simulink model "Calib_optitrack"  (R2024a)
settings: Solver=VariableStepAuto  StartTime=0.0  StopTime=10.0  RelTol=1e-3
libraries: robotcorelib x2
settings Model: Creator=user  LastModifiedBy=user

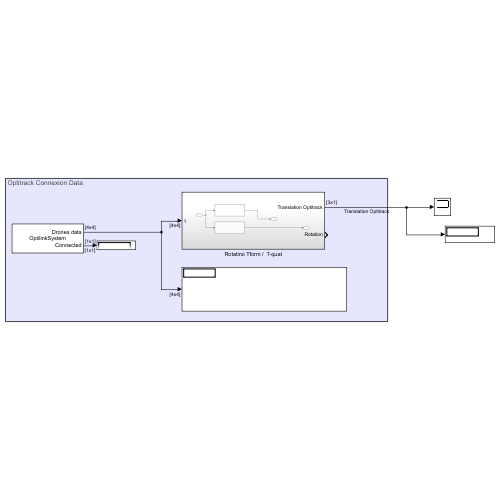
[thumbnail: Simulink's stored preview of the top-level diagram]
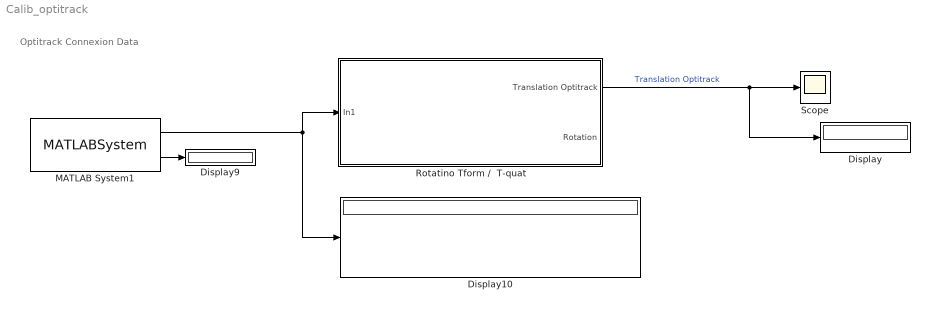
== system Calib_optitrack ==
  note: Optitrack Connexion Data
  Display : Display
  Display10 : Display
  Display9 : Display
  MATLAB System1 : MATLABSystem  System=OptilinkSystem  HostIP=127.0.0.1  ClientIP=127.0.0.1  SimulateUsing=Interpreted execution
      mask Type: OptilinkSystem
      mask Display:
      | disp('OptilinkSystem');
      | port_label('output',1,'Drones data');
      | port_label('output',2,'Connected');
  Rotatino Tform /  T-quat : Subsystem
  Scope : Scope
  wires:
  MATLAB System1/2 -> Display9/1
  Rotatino Tform /  T-quat/1(Translation Optitrack) -> Display/1, Scope/1  "Translation Optitrack"
  MATLAB System1/1 -> Rotatino Tform /  T-quat/1(In1), Display10/1

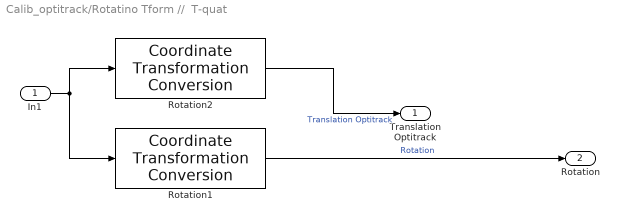
== system Calib_optitrack/Rotatino Tform //  T-quat ==
  In1 : Inport
  Rotation1 : robotcorelib/Coordinate Transformation Conversion  InputRepresentation=Homogeneous Transformation  InputEulerSequence=ZYX  ShowTrVecInputPort=on  OutputRepresentation=Quaternion  OutputEulerSequence=ZYX  ShowTrVecOutputPort=off  SimulateUsing=Code generation
      settings: LibrarySourceBlock=uavutilslib/Coordinate Transformation Conversion
  Rotation2 : robotcorelib/Coordinate Transformation Conversion  InputRepresentation=Homogeneous Transformation  InputEulerSequence=ZYX  ShowTrVecInputPort=on  OutputRepresentation=Translation Vector  OutputEulerSequence=ZYX  ShowTrVecOutputPort=off  SimulateUsing=Code generation
      settings: LibrarySourceBlock=uavutilslib/Coordinate Transformation Conversion
  Translation Optitrack : Outport
  Rotation : Outport  Port=2
  wires:
  Rotation1/1 -> Rotation/1  "Rotation"
  Rotation2/1 -> Translation Optitrack/1  "Translation Optitrack"
  In1/1 -> Rotation2/1, Rotation1/1
